simulink model "s12_euler_fvm_radiation_boundary_driver_ref"  (R2026a)
settings: Solver=FixedStepDiscrete  StartTime=0  StopTime=5.8309037900874641e-08  FixedStep=5.8309037900874641e-08
settings Model: Creator=Jovi  LastModifiedBy=Jovi

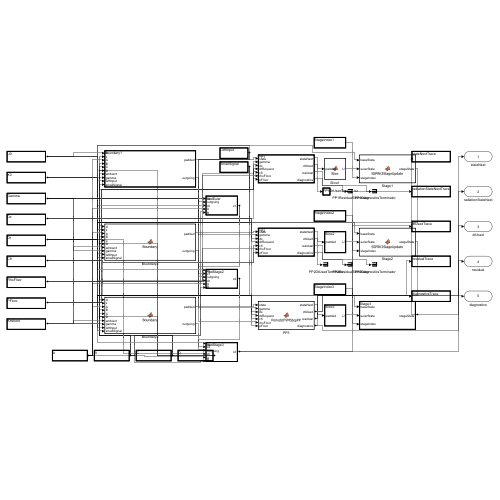
[thumbnail: Simulink's stored preview of the top-level diagram]
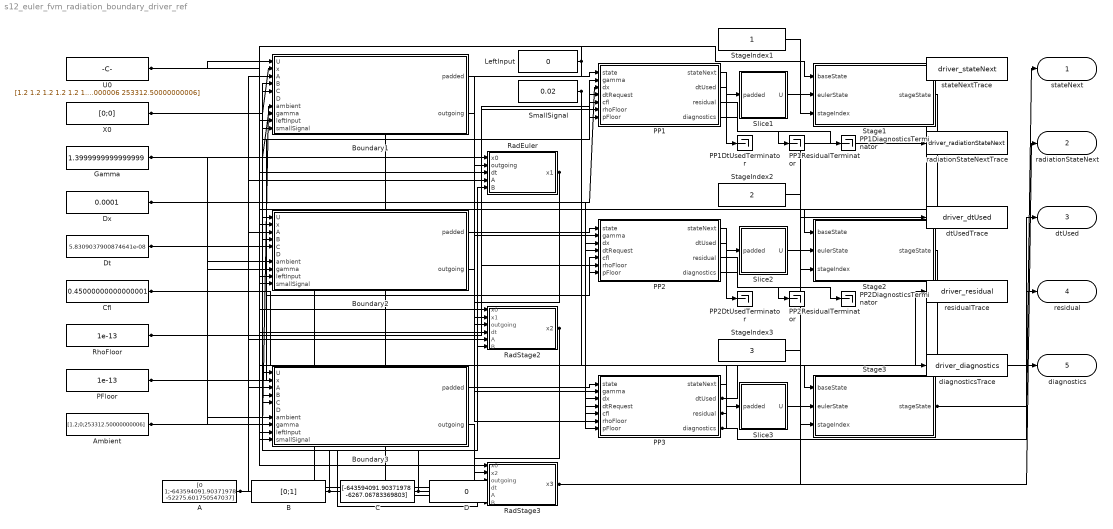
== system s12_euler_fvm_radiation_boundary_driver_ref ==
  A : Constant  Value=[0 1;-643594091.90371978 -52275.601750547037]  VectorParams1D=off  OutDataTypeStr=double
  Ambient : Constant  Value=[1.2;0;253312.50000000006]  VectorParams1D=off  OutDataTypeStr=double
  B : Constant  Value=[0;1]  VectorParams1D=off  OutDataTypeStr=double
  Boundary1 : MATLAB Function  TreatAsAtomicUnit=on
  Boundary2 : MATLAB Function  TreatAsAtomicUnit=on
  Boundary3 : MATLAB Function  TreatAsAtomicUnit=on
  C : Constant  Value=[-643594091.90371978 -6267.06783369803]  VectorParams1D=off  OutDataTypeStr=double
  Cfl : Constant  Value=0.45000000000000001  VectorParams1D=off  OutDataTypeStr=double
  D : Constant  Value=0  VectorParams1D=off  OutDataTypeStr=double
  Dt : Constant  Value=5.8309037900874641e-08  VectorParams1D=off  OutDataTypeStr=double
  Dx : Constant  Value=0.0001  VectorParams1D=off  OutDataTypeStr=double
  Gamma : Constant  Value=1.3999999999999999  VectorParams1D=off  OutDataTypeStr=double
  LeftInput : Constant  Value=0  VectorParams1D=off  OutDataTypeStr=double
  PFloor : Constant  Value=1e-13  VectorParams1D=off  OutDataTypeStr=double
  PP1 : MATLAB Function  TreatAsAtomicUnit=on
  PP1DiagnosticsTerminator : Terminator
  PP1DtUsedTerminator : Terminator
  PP1ResidualTerminator : Terminator
  PP2 : MATLAB Function  TreatAsAtomicUnit=on
  PP2DiagnosticsTerminator : Terminator
  PP2DtUsedTerminator : Terminator
  PP2ResidualTerminator : Terminator
  PP3 : MATLAB Function  TreatAsAtomicUnit=on
  RadEuler : MATLAB Function  TreatAsAtomicUnit=on
  RadStage2 : MATLAB Function  TreatAsAtomicUnit=on
  RadStage3 : MATLAB Function  TreatAsAtomicUnit=on
  RhoFloor : Constant  Value=1e-13  VectorParams1D=off  OutDataTypeStr=double
  Slice1 : MATLAB Function  TreatAsAtomicUnit=on
  Slice2 : MATLAB Function  TreatAsAtomicUnit=on
  Slice3 : MATLAB Function  TreatAsAtomicUnit=on
  SmallSignal : Constant  Value=0.02  VectorParams1D=off  OutDataTypeStr=double
  Stage1 : MATLAB Function  TreatAsAtomicUnit=on
  Stage2 : MATLAB Function  TreatAsAtomicUnit=on
  Stage3 : MATLAB Function  TreatAsAtomicUnit=on
  StageIndex1 : Constant  VectorParams1D=off  OutDataTypeStr=double
  StageIndex2 : Constant  Value=2  VectorParams1D=off  OutDataTypeStr=double
  StageIndex3 : Constant  Value=3  VectorParams1D=off  OutDataTypeStr=double
  U0 : Constant  Value=[1.2 1.2 1.2 1.2 1.2 1.2 1.2 1.2 1.2 1.2 1.2 1.2 1.2 1.2 1.2 1.2 1.2 1.2 1.2 1.2 1.2 1.2 1.2 1.2 1.2 1.2 1.2 1.2 1.2 1.2 1.2 1.2 1.2 1.2 1.2 1.2 1.2 1.2 1.2 1.2 1.2 1.2 1.2 1.2 1.2 1.2 1.2 1.2 1.2 1.2 1.2 1.2 1.2 1.2 1.2 1.2 1.2 1.2 1.2 1.2 1.2 1.2 1.2 1.2 1.2 1.2 1.2 1.2 1.2 1.2 1.2 1.2 1.2 1.2 1.2 1.2 1.2 1.2 1.2 1.2 1.2 1.2 1.2 1.2 1.2 1.2 1.2 1.2 1.2 1.2 1.2 1.2 1.2 1.2 1.2 1.2 1.2 1.2 1.2 1.2;0 0 0 0 0 0 0 0 0 0 0 0 0 0 0 0 0 0 0 0 0 0 0 0 0 0 0 0 0 0 0 0 0 0 0 0 0 0 0 0 0 0 0 0 0 0 0 0 0 0 0 0 0 0 0 0 0 0 0 0 0 0 0 0 0 0 0 0 0 0 0 0 0 0 0 0 0 0 0 0 0 0 0 0 0 0 0 0 0 0 0 0 0 0 0 0 0 0 0 0;253312.50000000006 253312.50000000006 253312.50000000006 253312.50000000006 253312.50000000006 253312.50000000006 253312.50000000006 253312.50000000006 253312.50000000006 253312.50000000006 253312.50000000006 253312.50000000006 253312.50000000006 253312.50000000006 253312.50000000006 253312.50000000006 253312.50000000006 253312.50000000006 253312.50000000006 253312.50000000006 253312.50000000006 253312.50000000006 253312.50000000006 253312.50000000006 253312.50000000006 253312.50000000006 253312.50000000006 253312.50000000006 253312.50000000006 253312.50000000006 253312.50000000006 253312.50000000006 253312.50000000006 253312.50000000006 253312.50000000006 253312.50000000006 253312.50000000006 253312.50000000006 253312.50000000006 253312.50000000006 253312.50000000006 253312.50000000006 253312.50000000006 253312.50000000006 253312.50000000006 253312.50000000006 253312.50000000006 253312.50000000006 253312.50000000006 253312.50000000006 253312.50000000006 253312.50000000006 253312.50000000006 253312.50000000006 253312.50000000006 253312.50000000006 253312.50000000006 253312.50000000006 253312.50000000006 253312.50000000006 253312.50000000006 253312.50000000006 253312.50000000006 253312.50000000006 253312.50000000006 253312.50000000006 253312.50000000006 253312.50000000006 253312.50000000006 253312.50000000006 253312.50000000006 253312.50000000006 253312.50000000006 253312.50000000006 253312.50000000006 253312.50000000006 253312.50000000006 253312.50000000006 253312.50000000006 253312.50000000006 253312.50000000006 253312.50000000006 253312.50000000006 253312.50000000006 253312.50000000006 253312.50000000006 253312.50000000006 253312.50000000006 253312.50000000006 253312.50000000006 253312.50000000006 253312.50000000006 253312.50000000006 253312.50000000006 253312.50000000006 253312.50000000006 253312.50000000006 253312.50000000006 253312.50000000006 253312.50000000006]  VectorParams1D=off  OutDataTypeStr=double
  X0 : Constant  Value=[0;0]  VectorParams1D=off  OutDataTypeStr=double
  diagnosticsTrace : ToWorkspace  VariableName=driver_diagnostics  SaveFormat=Structure With Time
      settings: MaxDataPoints=1
  dtUsedTrace : ToWorkspace  VariableName=driver_dtUsed  SaveFormat=Structure With Time
      settings: MaxDataPoints=1
  radiationStateNextTrace : ToWorkspace  VariableName=driver_radiationStateNext  SaveFormat=Structure With Time
      settings: MaxDataPoints=1
  residualTrace : ToWorkspace  VariableName=driver_residual  SaveFormat=Structure With Time
      settings: MaxDataPoints=1
  stateNextTrace : ToWorkspace  VariableName=driver_stateNext  SaveFormat=Structure With Time
      settings: MaxDataPoints=1
  stateNext : Outport
  radiationStateNext : Outport  Port=2
  dtUsed : Outport  Port=3
  residual : Outport  Port=4
  diagnostics : Outport  Port=5
  wires:
  U0/1 -> Boundary1/1(U), Stage1/1(baseState), Stage2/1(baseState), Stage3/1(baseState)
  X0/1 -> Boundary1/2(x), RadEuler/1(x0), RadStage2/1(x0), RadStage3/1(x0)
  A/1 -> Boundary1/3(A), RadEuler/4(A), Boundary2/3(A), RadStage2/5(A), Boundary3/3(A), RadStage3/5(A)
  B/1 -> Boundary1/4(B), RadEuler/5(B), Boundary2/4(B), RadStage2/6(B), Boundary3/4(B), RadStage3/6(B)
  C/1 -> Boundary1/5(C), Boundary2/5(C), Boundary3/5(C)
  D/1 -> Boundary1/6(D), Boundary2/6(D), Boundary3/6(D)
  Ambient/1 -> Boundary1/7(ambient), Boundary2/7(ambient), Boundary3/7(ambient)
  Gamma/1 -> Boundary1/8(gamma), PP1/2(gamma), Boundary2/8(gamma), PP2/2(gamma), Boundary3/8(gamma), PP3/2(gamma)
  LeftInput/1 -> Boundary1/9(leftInput), Boundary2/9(leftInput), Boundary3/9(leftInput)
  SmallSignal/1 -> Boundary1/10(smallSignal), Boundary2/10(smallSignal), Boundary3/10(smallSignal)
  Boundary1/1(padded) -> PP1/1(state)
  Dx/1 -> PP1/3(dx), PP2/3(dx), PP3/3(dx)
  Dt/1 -> PP1/4(dtRequest), RadEuler/3(dt), PP2/4(dtRequest), RadStage2/4(dt), PP3/4(dtRequest), RadStage3/4(dt)
  Cfl/1 -> PP1/5(cfl), PP2/5(cfl), PP3/5(cfl)
  RhoFloor/1 -> PP1/6(rhoFloor), PP2/6(rhoFloor), PP3/6(rhoFloor)
  PFloor/1 -> PP1/7(pFloor), PP2/7(pFloor), PP3/7(pFloor)
  PP1/1(stateNext) -> Slice1/1(padded)
  Slice1/1(U) -> Stage1/2(eulerState)
  StageIndex1/1 -> Stage1/3(stageIndex)
  Stage1/1(stageState) -> Boundary2/1(U)
  Boundary1/2(outgoing) -> RadEuler/2(outgoing)
  RadEuler/1(x1) -> Boundary2/2(x), RadStage2/2(x1)
  Boundary2/1(padded) -> PP2/1(state)
  PP2/1(stateNext) -> Slice2/1(padded)
  Slice2/1(U) -> Stage2/2(eulerState)
  StageIndex2/1 -> Stage2/3(stageIndex)
  Stage2/1(stageState) -> Boundary3/1(U)
  Boundary2/2(outgoing) -> RadStage2/3(outgoing)
  RadStage2/1(x2) -> Boundary3/2(x), RadStage3/2(x2)
  Boundary3/1(padded) -> PP3/1(state)
  PP3/1(stateNext) -> Slice3/1(padded)
  Slice3/1(U) -> Stage3/2(eulerState)
  StageIndex3/1 -> Stage3/3(stageIndex)
  Boundary3/2(outgoing) -> RadStage3/3(outgoing)
  Stage3/1(stageState) -> stateNext/1, stateNextTrace/1
  RadStage3/1(x3) -> radiationStateNext/1, radiationStateNextTrace/1
  PP3/2(dtUsed) -> dtUsed/1, dtUsedTrace/1
  PP3/3(residual) -> residual/1, residualTrace/1
  PP3/4(diagnostics) -> diagnostics/1, diagnosticsTrace/1
  PP1/2(dtUsed) -> PP1DtUsedTerminator/1
  PP1/3(residual) -> PP1ResidualTerminator/1
  PP1/4(diagnostics) -> PP1DiagnosticsTerminator/1
  PP2/2(dtUsed) -> PP2DtUsedTerminator/1
  PP2/3(residual) -> PP2ResidualTerminator/1
  PP2/4(diagnostics) -> PP2DiagnosticsTerminator/1

== matlab function s12_euler_fvm_radiation_boundary_driver_ref/Boundary2 ==
  data: U input; padded output; x input; A input; B input; C input; D input; ambient input; gamma input; leftInput input; smallSignal input; outgoing output
function [padded,outgoing] = Boundary(U,x,A,B,C,D,ambient,gamma,leftInput,smallSignal)
%#codegen
padded = zeros(3,size(U,2)+4); outgoing = 0;
[rho,u,p] = primitive(U(:,end),gamma); %#ok<ASGLU>
[rho0,u0,p0,c0] = primitive(ambient,gamma); %#ok<ASGLU>
outgoing = 0.5*((p-p0)+rho0*c0*u);
incoming = C*x + D*outgoing; perturbation = outgoing + incoming;
if max(abs([outgoing,incoming,perturbation])) > smallSignal*p0, error('S12:Driver:SmallSignal', 'Radiation boundary perturbation exceeds the configured small-signal limit.'); end
boundaryPressure = p0 + perturbation;
boundaryDensity = rho0 + perturbation/c0^2;
boundaryVelocity = (outgoing-incoming)/(rho0*c0);
right = conservative(boundaryDensity,boundaryVelocity,boundaryPressure,gamma);
left = leftBoundary(U(:,1),ambient,gamma,leftInput,smallSignal);
padded(:,1)=left; padded(:,2)=left; padded(:,3:end-2)=U; padded(:,end-1)=right; padded(:,end)=right;
end
function state = leftBoundary(interior,ambient,gamma,incomingPressure,smallSignal)
if all(interior == ambient), state=interior; return; end
[rho,u,p,c] = primitive(interior,gamma); [rho0,u0,p0,c0] = primitive(ambient,gamma);
if abs(incomingPressure) > smallSignal*p0, error('S12:Driver:SmallSignal', 'Radiation boundary perturbation exceeds the configured small-signal limit.'); end
if abs(incomingPressure) > 0
outgoing = 0.5*((p-p0)-rho0*c0*u); boundaryPressure=p0+incomingPressure+outgoing; boundaryVelocity=(incomingPressure-outgoing)/(rho0*c0); boundaryDensity=rho0*(boundaryPressure/p0)^(1/gamma);
else
incomingAmbient=u0+2*c0/(gamma-1); outgoing=u-2*c/(gamma-1); boundaryVelocity=0.5*(outgoing+incomingAmbient); boundarySoundSpeed=0.25*(gamma-1)*(incomingAmbient-outgoing); entropy=p/rho^gamma; boundaryDensity=(boundarySoundSpeed^2/(gamma*entropy))^(1/(gamma-1)); boundaryPressure=entropy*boundaryDensity^gamma;
end
state=conservative(boundaryDensity,boundaryVelocity,boundaryPressure,gamma);
end
function [rho,u,p,c] = primitive(state,gamma)
rho=state(1); u=state(2)/rho; p=(gamma-1)*(state(3)-0.5*rho*u^2); c=sqrt(gamma*p/rho);
end
function state=conservative(rho,u,p,gamma)
state=[rho;rho*u;p/(gamma-1)+0.5*rho*u^2];
end

== matlab function s12_euler_fvm_radiation_boundary_driver_ref/Boundary3 ==
  data: U input; padded output; x input; A input; B input; C input; D input; ambient input; gamma input; leftInput input; smallSignal input; outgoing output
function [padded,outgoing] = Boundary(U,x,A,B,C,D,ambient,gamma,leftInput,smallSignal)
%#codegen
padded = zeros(3,size(U,2)+4); outgoing = 0;
[rho,u,p] = primitive(U(:,end),gamma); %#ok<ASGLU>
[rho0,u0,p0,c0] = primitive(ambient,gamma); %#ok<ASGLU>
outgoing = 0.5*((p-p0)+rho0*c0*u);
incoming = C*x + D*outgoing; perturbation = outgoing + incoming;
if max(abs([outgoing,incoming,perturbation])) > smallSignal*p0, error('S12:Driver:SmallSignal', 'Radiation boundary perturbation exceeds the configured small-signal limit.'); end
boundaryPressure = p0 + perturbation;
boundaryDensity = rho0 + perturbation/c0^2;
boundaryVelocity = (outgoing-incoming)/(rho0*c0);
right = conservative(boundaryDensity,boundaryVelocity,boundaryPressure,gamma);
left = leftBoundary(U(:,1),ambient,gamma,leftInput,smallSignal);
padded(:,1)=left; padded(:,2)=left; padded(:,3:end-2)=U; padded(:,end-1)=right; padded(:,end)=right;
end
function state = leftBoundary(interior,ambient,gamma,incomingPressure,smallSignal)
if all(interior == ambient), state=interior; return; end
[rho,u,p,c] = primitive(interior,gamma); [rho0,u0,p0,c0] = primitive(ambient,gamma);
if abs(incomingPressure) > smallSignal*p0, error('S12:Driver:SmallSignal', 'Radiation boundary perturbation exceeds the configured small-signal limit.'); end
if abs(incomingPressure) > 0
outgoing = 0.5*((p-p0)-rho0*c0*u); boundaryPressure=p0+incomingPressure+outgoing; boundaryVelocity=(incomingPressure-outgoing)/(rho0*c0); boundaryDensity=rho0*(boundaryPressure/p0)^(1/gamma);
else
incomingAmbient=u0+2*c0/(gamma-1); outgoing=u-2*c/(gamma-1); boundaryVelocity=0.5*(outgoing+incomingAmbient); boundarySoundSpeed=0.25*(gamma-1)*(incomingAmbient-outgoing); entropy=p/rho^gamma; boundaryDensity=(boundarySoundSpeed^2/(gamma*entropy))^(1/(gamma-1)); boundaryPressure=entropy*boundaryDensity^gamma;
end
state=conservative(boundaryDensity,boundaryVelocity,boundaryPressure,gamma);
end
function [rho,u,p,c] = primitive(state,gamma)
rho=state(1); u=state(2)/rho; p=(gamma-1)*(state(3)-0.5*rho*u^2); c=sqrt(gamma*p/rho);
end
function state=conservative(rho,u,p,gamma)
state=[rho;rho*u;p/(gamma-1)+0.5*rho*u^2];
end

== matlab function s12_euler_fvm_radiation_boundary_driver_ref/Slice1 ==
  data: padded input; U output
function U = Slice(padded)
%#codegen
U=zeros(3,size(padded,2)-4); U(:,:)=padded(:,3:end-2);
end

== matlab function s12_euler_fvm_radiation_boundary_driver_ref/Slice2 ==
  data: padded input; U output
function U = Slice(padded)
%#codegen
U=zeros(3,size(padded,2)-4); U(:,:)=padded(:,3:end-2);
end

== matlab function s12_euler_fvm_radiation_boundary_driver_ref/Slice3 ==
  data: padded input; U output
function U = Slice(padded)
%#codegen
U=zeros(3,size(padded,2)-4); U(:,:)=padded(:,3:end-2);
end

== matlab function s12_euler_fvm_radiation_boundary_driver_ref/RadEuler ==
  data: x0 input; x1 output; outgoing input; dt input; A input; B input
function x1 = RadEuler(x0,outgoing,dt,A,B)
%#codegen
x1=zeros(2,1); x1=x0+dt*(A*x0+B*outgoing);
end

== matlab function s12_euler_fvm_radiation_boundary_driver_ref/PP2 ==
  data: state input; stateNext output; gamma input; dx input; dtRequest input; cfl input; dtUsed output; residual output; rhoFloor input; pFloor input; diagnostics output
function [stateNext,dtUsed,residual,diagnostics] = PeriodicFVMStepPP(state,gamma,dx,dtRequest,cfl,rhoFloor,pFloor)
%#codegen
validateState(state,gamma,rhoFloor,pFloor);
cellCount = size(state,2);
alphaStage = stageAlpha(state,gamma);
dtUsed = min(dtRequest,cfl*dx/alphaStage);
lambda = dtUsed/dx;
[rho,velocity,pressure] = recoverPrimitives(state,gamma);
slopeRho = minmodSlopes(rho);
slopeVelocity = minmodSlopes(velocity);
slopePressure = minmodSlopes(pressure);
leftPrimitive = zeros(3,cellCount);
rightPrimitive = zeros(3,cellCount);
minmodActivationCount = 0;
minmodLimitedCellCount = 0;
reconstructionPPActivationCount = 0;
reconstructionPPLimitedCellCount = 0;
reconstructionPPMinTheta = 1;
minimumReconstructedDensity = inf;
minimumReconstructedPressure = inf;
for cellIndex = 1:cellCount
    leftIndex = mod(cellIndex-2,cellCount)+1;
    rightIndex = mod(cellIndex,cellCount)+1;
    centered = 0.5*[rho(rightIndex)-rho(leftIndex);velocity(rightIndex)-velocity(leftIndex);pressure(rightIndex)-pressure(leftIndex)];
    slopes = [slopeRho(cellIndex);slopeVelocity(cellIndex);slopePressure(cellIndex)];
    limited = abs(slopes-centered) > 32*eps(max([1;abs(slopes);abs(centered)]));
    minmodActivationCount = minmodActivationCount + sum(limited);
    minmodLimitedCellCount = minmodLimitedCellCount + double(any(limited));
    primitive = [rho(cellIndex);velocity(cellIndex);pressure(cellIndex)];
    reconstruction = s12_pp_reconstruct_primitive(primitive,slopes,rhoFloor,pFloor);
    leftPrimitive(:,cellIndex) = reconstruction.left;
    rightPrimitive(:,cellIndex) = reconstruction.right;
    reconstructionPPMinTheta = min(reconstructionPPMinTheta,reconstruction.theta);
    active = reconstruction.theta < 1-32*eps;
    reconstructionPPActivationCount = reconstructionPPActivationCount + double(active);
    reconstructionPPLimitedCellCount = reconstructionPPLimitedCellCount + double(active);
    minimumReconstructedDensity = min(minimumReconstructedDensity,min(reconstruction.left(1),reconstruction.right(1)));
    minimumReconstructedPressure = min(minimumReconstructedPressure,min(reconstruction.left(3),reconstruction.right(3)));
end
interfaceFlux = zeros(3,cellCount);
fluxPPActivationCount = 0;
fluxPPLimitedInterfaceCount = 0;
fluxPPMinTheta = 1;
minimumAnchorDensity = inf;
minimumAnchorPressure = inf;
minimumFinalPartialDensity = inf;
minimumFinalPartialPressure = inf;
maximumFluxCorrectionNorm = 0;
for interfaceIndex = 1:cellCount
    rightIndex = mod(interfaceIndex,cellCount)+1;
    leftState = conservativeFromPrimitives(rightPrimitive(1,interfaceIndex),rightPrimitive(2,interfaceIndex),rightPrimitive(3,interfaceIndex),gamma);
    rightState = conservativeFromPrimitives(leftPrimitive(1,rightIndex),leftPrimitive(2,rightIndex),leftPrimitive(3,rightIndex),gamma);
    highFlux = hllcFlux(leftState,rightState,gamma);
    lowFlux = s12_pp_global_lf_flux(state(:,interfaceIndex),state(:,rightIndex),gamma,alphaStage);
    limitedFlux = s12_pp_limit_interface_flux(state(:,interfaceIndex),state(:,rightIndex),highFlux,lowFlux,lambda,gamma,rhoFloor,pFloor);
    interfaceFlux(:,interfaceIndex) = limitedFlux.flux;
    fluxPPMinTheta = min(fluxPPMinTheta,limitedFlux.theta);
    active = limitedFlux.theta < 1-32*eps;
    fluxPPActivationCount = fluxPPActivationCount + double(active);
    fluxPPLimitedInterfaceCount = fluxPPLimitedInterfaceCount + double(active);
    minimumAnchorDensity = min(minimumAnchorDensity,min(limitedFlux.low_left_partial(1),limitedFlux.low_right_partial(1)));
    minimumAnchorPressure = min(minimumAnchorPressure,min(pressureOf(limitedFlux.low_left_partial,gamma),pressureOf(limitedFlux.low_right_partial,gamma)));
    minimumFinalPartialDensity = min(minimumFinalPartialDensity,min(limitedFlux.left_partial(1),limitedFlux.right_partial(1)));
    minimumFinalPartialPressure = min(minimumFinalPartialPressure,min(pressureOf(limitedFlux.left_partial,gamma),pressureOf(limitedFlux.right_partial,gamma)));
    maximumFluxCorrectionNorm = max(maximumFluxCorrectionNorm,limitedFlux.correction_norm);
end
stateNext = zeros(size(state));
for cellIndex = 1:cellCount
    leftInterface = mod(cellIndex-2,cellCount)+1;
    stateNext(:,cellIndex) = state(:,cellIndex)-lambda*(interfaceFlux(:,cellIndex)-interfaceFlux(:,leftInterface));
end
validateState(stateNext,gamma,rhoFloor,pFloor);
residual = sum(stateNext-state,2).';
diagnostics = [minmodActivationCount,minmodLimitedCellCount,cellCount,reconstructionPPActivationCount,reconstructionPPLimitedCellCount,reconstructionPPMinTheta,minimumReconstructedDensity,minimumReconstructedPressure,0,fluxPPActivationCount,fluxPPLimitedInterfaceCount,cellCount,fluxPPMinTheta,minimumAnchorDensity,minimumAnchorPressure,minimumFinalPartialDensity,minimumFinalPartialPressure,alphaStage,maximumFluxCorrectionNorm,0];
end

function alpha = stageAlpha(state,gamma)
[rho,velocity,pressure] = recoverPrimitives(state,gamma);
alpha = max(abs(velocity)+sqrt(gamma*pressure./rho));
end

function validateState(state,gamma,rhoFloor,pFloor)
[rho,~,pressure] = recoverPrimitives(state,gamma);
if any(~isfinite(state(:))) || any(rho < rhoFloor) || any(pressure < pFloor)
    error('S12:Positivity:InvalidStage','A PP stage violated the configured floors.');
end
end

function [rho,velocity,pressure] = recoverPrimitives(state,gamma)
rho = state(1,:);
velocity = state(2,:)./rho;
pressure = (gamma-1)*(state(3,:)-0.5*rho.*velocity.^2);
end

function value = pressureOf(state,gamma)
rho = state(1);
velocity = state(2)/rho;
value = (gamma-1)*(state(3)-0.5*rho*velocity^2);
end

function state = conservativeFromPrimitives(rho,velocity,pressure,gamma)
state = [rho;rho*velocity;pressure/(gamma-1)+0.5*rho*velocity^2];
end

function slopes = minmodSlopes(values)
cellCount = numel(values);
slopes = zeros(size(values));
for cellIndex = 1:cellCount
    leftIndex = mod(cellIndex-2,cellCount)+1;
    rightIndex = mod(cellIndex,cellCount)+1;
    slopes(cellIndex) = minmod(values(cellIndex)-values(leftIndex),values(rightIndex)-values(cellIndex));
end
end

function value = minmod(leftDelta,rightDelta)
if leftDelta*rightDelta <= 0
    value = 0;
elseif abs(leftDelta) <= abs(rightDelta)
    value = leftDelta;
else
    value = rightDelta;
end
end

function flux = hllcFlux(stateL,stateR,gamma)
rhoL = stateL(1); rhoR = stateR(1);
uL = stateL(2)/rhoL; uR = stateR(2)/rhoR;
energyL = stateL(3); energyR = stateR(3);
pL = (gamma-1)*(energyL-0.5*rhoL*uL*uL);
pR = (gamma-1)*(energyR-0.5*rhoR*uR*uR);
soundL = sqrt(gamma*pL/rhoL); soundR = sqrt(gamma*pR/rhoR);
sL = min(uL-soundL,uR-soundR); sR = max(uL+soundL,uR+soundR);
sM = (pR-pL+rhoL*uL*(sL-uL)-rhoR*uR*(sR-uR))/(rhoL*(sL-uL)-rhoR*(sR-uR));
fluxL = [rhoL*uL;rhoL*uL*uL+pL;uL*(energyL+pL)];
fluxR = [rhoR*uR;rhoR*uR*uR+pR;uR*(energyR+pR)];
if sL >= 0
    flux = fluxL;
elseif sM >= 0
    rhoStarL = rhoL*(sL-uL)/(sL-sM);
    energyStarL = rhoStarL*(energyL/rhoL+(sM-uL)*(sM+pL/(rhoL*(sL-uL))));
    flux = fluxL+sL*([rhoStarL;rhoStarL*sM;energyStarL]-stateL);
elseif sR > 0
    rhoStarR = rhoR*(sR-uR)/(sR-sM);
    energyStarR = rhoStarR*(energyR/rhoR+(sM-uR)*(sM+pR/(rhoR*(sR-uR))));
    flux = fluxR+sR*([rhoStarR;rhoStarR*sM;energyStarR]-stateR);
else
    flux = fluxR;
end
end

== matlab function s12_euler_fvm_radiation_boundary_driver_ref/RadStage2 ==
  data: x0 input; x2 output; x1 input; outgoing input; dt input; A input; B input
function x2 = RadStage2(x0,x1,outgoing,dt,A,B)
%#codegen
x2=zeros(2,1); x2=0.75*x0+0.25*(x1+dt*(A*x1+B*outgoing));
end

== matlab function s12_euler_fvm_radiation_boundary_driver_ref/RadStage3 ==
  data: x0 input; x3 output; x2 input; outgoing input; dt input; A input; B input
function x3 = RadStage3(x0,x2,outgoing,dt,A,B)
%#codegen
x3=zeros(2,1); x3=(1/3)*x0+(2/3)*(x2+dt*(A*x2+B*outgoing));
end

== matlab function s12_euler_fvm_radiation_boundary_driver_ref/PP1 ==
  data: state input; stateNext output; gamma input; dx input; dtRequest input; cfl input; dtUsed output; residual output; rhoFloor input; pFloor input; diagnostics output
function [stateNext,dtUsed,residual,diagnostics] = PeriodicFVMStepPP(state,gamma,dx,dtRequest,cfl,rhoFloor,pFloor)
%#codegen
validateState(state,gamma,rhoFloor,pFloor);
cellCount = size(state,2);
alphaStage = stageAlpha(state,gamma);
dtUsed = min(dtRequest,cfl*dx/alphaStage);
lambda = dtUsed/dx;
[rho,velocity,pressure] = recoverPrimitives(state,gamma);
slopeRho = minmodSlopes(rho);
slopeVelocity = minmodSlopes(velocity);
slopePressure = minmodSlopes(pressure);
leftPrimitive = zeros(3,cellCount);
rightPrimitive = zeros(3,cellCount);
minmodActivationCount = 0;
minmodLimitedCellCount = 0;
reconstructionPPActivationCount = 0;
reconstructionPPLimitedCellCount = 0;
reconstructionPPMinTheta = 1;
minimumReconstructedDensity = inf;
minimumReconstructedPressure = inf;
for cellIndex = 1:cellCount
    leftIndex = mod(cellIndex-2,cellCount)+1;
    rightIndex = mod(cellIndex,cellCount)+1;
    centered = 0.5*[rho(rightIndex)-rho(leftIndex);velocity(rightIndex)-velocity(leftIndex);pressure(rightIndex)-pressure(leftIndex)];
    slopes = [slopeRho(cellIndex);slopeVelocity(cellIndex);slopePressure(cellIndex)];
    limited = abs(slopes-centered) > 32*eps(max([1;abs(slopes);abs(centered)]));
    minmodActivationCount = minmodActivationCount + sum(limited);
    minmodLimitedCellCount = minmodLimitedCellCount + double(any(limited));
    primitive = [rho(cellIndex);velocity(cellIndex);pressure(cellIndex)];
    reconstruction = s12_pp_reconstruct_primitive(primitive,slopes,rhoFloor,pFloor);
    leftPrimitive(:,cellIndex) = reconstruction.left;
    rightPrimitive(:,cellIndex) = reconstruction.right;
    reconstructionPPMinTheta = min(reconstructionPPMinTheta,reconstruction.theta);
    active = reconstruction.theta < 1-32*eps;
    reconstructionPPActivationCount = reconstructionPPActivationCount + double(active);
    reconstructionPPLimitedCellCount = reconstructionPPLimitedCellCount + double(active);
    minimumReconstructedDensity = min(minimumReconstructedDensity,min(reconstruction.left(1),reconstruction.right(1)));
    minimumReconstructedPressure = min(minimumReconstructedPressure,min(reconstruction.left(3),reconstruction.right(3)));
end
interfaceFlux = zeros(3,cellCount);
fluxPPActivationCount = 0;
fluxPPLimitedInterfaceCount = 0;
fluxPPMinTheta = 1;
minimumAnchorDensity = inf;
minimumAnchorPressure = inf;
minimumFinalPartialDensity = inf;
minimumFinalPartialPressure = inf;
maximumFluxCorrectionNorm = 0;
for interfaceIndex = 1:cellCount
    rightIndex = mod(interfaceIndex,cellCount)+1;
    leftState = conservativeFromPrimitives(rightPrimitive(1,interfaceIndex),rightPrimitive(2,interfaceIndex),rightPrimitive(3,interfaceIndex),gamma);
    rightState = conservativeFromPrimitives(leftPrimitive(1,rightIndex),leftPrimitive(2,rightIndex),leftPrimitive(3,rightIndex),gamma);
    highFlux = hllcFlux(leftState,rightState,gamma);
    lowFlux = s12_pp_global_lf_flux(state(:,interfaceIndex),state(:,rightIndex),gamma,alphaStage);
    limitedFlux = s12_pp_limit_interface_flux(state(:,interfaceIndex),state(:,rightIndex),highFlux,lowFlux,lambda,gamma,rhoFloor,pFloor);
    interfaceFlux(:,interfaceIndex) = limitedFlux.flux;
    fluxPPMinTheta = min(fluxPPMinTheta,limitedFlux.theta);
    active = limitedFlux.theta < 1-32*eps;
    fluxPPActivationCount = fluxPPActivationCount + double(active);
    fluxPPLimitedInterfaceCount = fluxPPLimitedInterfaceCount + double(active);
    minimumAnchorDensity = min(minimumAnchorDensity,min(limitedFlux.low_left_partial(1),limitedFlux.low_right_partial(1)));
    minimumAnchorPressure = min(minimumAnchorPressure,min(pressureOf(limitedFlux.low_left_partial,gamma),pressureOf(limitedFlux.low_right_partial,gamma)));
    minimumFinalPartialDensity = min(minimumFinalPartialDensity,min(limitedFlux.left_partial(1),limitedFlux.right_partial(1)));
    minimumFinalPartialPressure = min(minimumFinalPartialPressure,min(pressureOf(limitedFlux.left_partial,gamma),pressureOf(limitedFlux.right_partial,gamma)));
    maximumFluxCorrectionNorm = max(maximumFluxCorrectionNorm,limitedFlux.correction_norm);
end
stateNext = zeros(size(state));
for cellIndex = 1:cellCount
    leftInterface = mod(cellIndex-2,cellCount)+1;
    stateNext(:,cellIndex) = state(:,cellIndex)-lambda*(interfaceFlux(:,cellIndex)-interfaceFlux(:,leftInterface));
end
validateState(stateNext,gamma,rhoFloor,pFloor);
residual = sum(stateNext-state,2).';
diagnostics = [minmodActivationCount,minmodLimitedCellCount,cellCount,reconstructionPPActivationCount,reconstructionPPLimitedCellCount,reconstructionPPMinTheta,minimumReconstructedDensity,minimumReconstructedPressure,0,fluxPPActivationCount,fluxPPLimitedInterfaceCount,cellCount,fluxPPMinTheta,minimumAnchorDensity,minimumAnchorPressure,minimumFinalPartialDensity,minimumFinalPartialPressure,alphaStage,maximumFluxCorrectionNorm,0];
end

function alpha = stageAlpha(state,gamma)
[rho,velocity,pressure] = recoverPrimitives(state,gamma);
alpha = max(abs(velocity)+sqrt(gamma*pressure./rho));
end

function validateState(state,gamma,rhoFloor,pFloor)
[rho,~,pressure] = recoverPrimitives(state,gamma);
if any(~isfinite(state(:))) || any(rho < rhoFloor) || any(pressure < pFloor)
    error('S12:Positivity:InvalidStage','A PP stage violated the configured floors.');
end
end

function [rho,velocity,pressure] = recoverPrimitives(state,gamma)
rho = state(1,:);
velocity = state(2,:)./rho;
pressure = (gamma-1)*(state(3,:)-0.5*rho.*velocity.^2);
end

function value = pressureOf(state,gamma)
rho = state(1);
velocity = state(2)/rho;
value = (gamma-1)*(state(3)-0.5*rho*velocity^2);
end

function state = conservativeFromPrimitives(rho,velocity,pressure,gamma)
state = [rho;rho*velocity;pressure/(gamma-1)+0.5*rho*velocity^2];
end

function slopes = minmodSlopes(values)
cellCount = numel(values);
slopes = zeros(size(values));
for cellIndex = 1:cellCount
    leftIndex = mod(cellIndex-2,cellCount)+1;
    rightIndex = mod(cellIndex,cellCount)+1;
    slopes(cellIndex) = minmod(values(cellIndex)-values(leftIndex),values(rightIndex)-values(cellIndex));
end
end

function value = minmod(leftDelta,rightDelta)
if leftDelta*rightDelta <= 0
    value = 0;
elseif abs(leftDelta) <= abs(rightDelta)
    value = leftDelta;
else
    value = rightDelta;
end
end

function flux = hllcFlux(stateL,stateR,gamma)
rhoL = stateL(1); rhoR = stateR(1);
uL = stateL(2)/rhoL; uR = stateR(2)/rhoR;
energyL = stateL(3); energyR = stateR(3);
pL = (gamma-1)*(energyL-0.5*rhoL*uL*uL);
pR = (gamma-1)*(energyR-0.5*rhoR*uR*uR);
soundL = sqrt(gamma*pL/rhoL); soundR = sqrt(gamma*pR/rhoR);
sL = min(uL-soundL,uR-soundR); sR = max(uL+soundL,uR+soundR);
sM = (pR-pL+rhoL*uL*(sL-uL)-rhoR*uR*(sR-uR))/(rhoL*(sL-uL)-rhoR*(sR-uR));
fluxL = [rhoL*uL;rhoL*uL*uL+pL;uL*(energyL+pL)];
fluxR = [rhoR*uR;rhoR*uR*uR+pR;uR*(energyR+pR)];
if sL >= 0
    flux = fluxL;
elseif sM >= 0
    rhoStarL = rhoL*(sL-uL)/(sL-sM);
    energyStarL = rhoStarL*(energyL/rhoL+(sM-uL)*(sM+pL/(rhoL*(sL-uL))));
    flux = fluxL+sL*([rhoStarL;rhoStarL*sM;energyStarL]-stateL);
elseif sR > 0
    rhoStarR = rhoR*(sR-uR)/(sR-sM);
    energyStarR = rhoStarR*(energyR/rhoR+(sM-uR)*(sM+pR/(rhoR*(sR-uR))));
    flux = fluxR+sR*([rhoStarR;rhoStarR*sM;energyStarR]-stateR);
else
    flux = fluxR;
end
end

== matlab function s12_euler_fvm_radiation_boundary_driver_ref/PP3 ==
  data: state input; stateNext output; gamma input; dx input; dtRequest input; cfl input; dtUsed output; residual output; rhoFloor input; pFloor input; diagnostics output
function [stateNext,dtUsed,residual,diagnostics] = PeriodicFVMStepPP(state,gamma,dx,dtRequest,cfl,rhoFloor,pFloor)
%#codegen
validateState(state,gamma,rhoFloor,pFloor);
cellCount = size(state,2);
alphaStage = stageAlpha(state,gamma);
dtUsed = min(dtRequest,cfl*dx/alphaStage);
lambda = dtUsed/dx;
[rho,velocity,pressure] = recoverPrimitives(state,gamma);
slopeRho = minmodSlopes(rho);
slopeVelocity = minmodSlopes(velocity);
slopePressure = minmodSlopes(pressure);
leftPrimitive = zeros(3,cellCount);
rightPrimitive = zeros(3,cellCount);
minmodActivationCount = 0;
minmodLimitedCellCount = 0;
reconstructionPPActivationCount = 0;
reconstructionPPLimitedCellCount = 0;
reconstructionPPMinTheta = 1;
minimumReconstructedDensity = inf;
minimumReconstructedPressure = inf;
for cellIndex = 1:cellCount
    leftIndex = mod(cellIndex-2,cellCount)+1;
    rightIndex = mod(cellIndex,cellCount)+1;
    centered = 0.5*[rho(rightIndex)-rho(leftIndex);velocity(rightIndex)-velocity(leftIndex);pressure(rightIndex)-pressure(leftIndex)];
    slopes = [slopeRho(cellIndex);slopeVelocity(cellIndex);slopePressure(cellIndex)];
    limited = abs(slopes-centered) > 32*eps(max([1;abs(slopes);abs(centered)]));
    minmodActivationCount = minmodActivationCount + sum(limited);
    minmodLimitedCellCount = minmodLimitedCellCount + double(any(limited));
    primitive = [rho(cellIndex);velocity(cellIndex);pressure(cellIndex)];
    reconstruction = s12_pp_reconstruct_primitive(primitive,slopes,rhoFloor,pFloor);
    leftPrimitive(:,cellIndex) = reconstruction.left;
    rightPrimitive(:,cellIndex) = reconstruction.right;
    reconstructionPPMinTheta = min(reconstructionPPMinTheta,reconstruction.theta);
    active = reconstruction.theta < 1-32*eps;
    reconstructionPPActivationCount = reconstructionPPActivationCount + double(active);
    reconstructionPPLimitedCellCount = reconstructionPPLimitedCellCount + double(active);
    minimumReconstructedDensity = min(minimumReconstructedDensity,min(reconstruction.left(1),reconstruction.right(1)));
    minimumReconstructedPressure = min(minimumReconstructedPressure,min(reconstruction.left(3),reconstruction.right(3)));
end
interfaceFlux = zeros(3,cellCount);
fluxPPActivationCount = 0;
fluxPPLimitedInterfaceCount = 0;
fluxPPMinTheta = 1;
minimumAnchorDensity = inf;
minimumAnchorPressure = inf;
minimumFinalPartialDensity = inf;
minimumFinalPartialPressure = inf;
maximumFluxCorrectionNorm = 0;
for interfaceIndex = 1:cellCount
    rightIndex = mod(interfaceIndex,cellCount)+1;
    leftState = conservativeFromPrimitives(rightPrimitive(1,interfaceIndex),rightPrimitive(2,interfaceIndex),rightPrimitive(3,interfaceIndex),gamma);
    rightState = conservativeFromPrimitives(leftPrimitive(1,rightIndex),leftPrimitive(2,rightIndex),leftPrimitive(3,rightIndex),gamma);
    highFlux = hllcFlux(leftState,rightState,gamma);
    lowFlux = s12_pp_global_lf_flux(state(:,interfaceIndex),state(:,rightIndex),gamma,alphaStage);
    limitedFlux = s12_pp_limit_interface_flux(state(:,interfaceIndex),state(:,rightIndex),highFlux,lowFlux,lambda,gamma,rhoFloor,pFloor);
    interfaceFlux(:,interfaceIndex) = limitedFlux.flux;
    fluxPPMinTheta = min(fluxPPMinTheta,limitedFlux.theta);
    active = limitedFlux.theta < 1-32*eps;
    fluxPPActivationCount = fluxPPActivationCount + double(active);
    fluxPPLimitedInterfaceCount = fluxPPLimitedInterfaceCount + double(active);
    minimumAnchorDensity = min(minimumAnchorDensity,min(limitedFlux.low_left_partial(1),limitedFlux.low_right_partial(1)));
    minimumAnchorPressure = min(minimumAnchorPressure,min(pressureOf(limitedFlux.low_left_partial,gamma),pressureOf(limitedFlux.low_right_partial,gamma)));
    minimumFinalPartialDensity = min(minimumFinalPartialDensity,min(limitedFlux.left_partial(1),limitedFlux.right_partial(1)));
    minimumFinalPartialPressure = min(minimumFinalPartialPressure,min(pressureOf(limitedFlux.left_partial,gamma),pressureOf(limitedFlux.right_partial,gamma)));
    maximumFluxCorrectionNorm = max(maximumFluxCorrectionNorm,limitedFlux.correction_norm);
end
stateNext = zeros(size(state));
for cellIndex = 1:cellCount
    leftInterface = mod(cellIndex-2,cellCount)+1;
    stateNext(:,cellIndex) = state(:,cellIndex)-lambda*(interfaceFlux(:,cellIndex)-interfaceFlux(:,leftInterface));
end
validateState(stateNext,gamma,rhoFloor,pFloor);
residual = sum(stateNext-state,2).';
diagnostics = [minmodActivationCount,minmodLimitedCellCount,cellCount,reconstructionPPActivationCount,reconstructionPPLimitedCellCount,reconstructionPPMinTheta,minimumReconstructedDensity,minimumReconstructedPressure,0,fluxPPActivationCount,fluxPPLimitedInterfaceCount,cellCount,fluxPPMinTheta,minimumAnchorDensity,minimumAnchorPressure,minimumFinalPartialDensity,minimumFinalPartialPressure,alphaStage,maximumFluxCorrectionNorm,0];
end

function alpha = stageAlpha(state,gamma)
[rho,velocity,pressure] = recoverPrimitives(state,gamma);
alpha = max(abs(velocity)+sqrt(gamma*pressure./rho));
end

function validateState(state,gamma,rhoFloor,pFloor)
[rho,~,pressure] = recoverPrimitives(state,gamma);
if any(~isfinite(state(:))) || any(rho < rhoFloor) || any(pressure < pFloor)
    error('S12:Positivity:InvalidStage','A PP stage violated the configured floors.');
end
end

function [rho,velocity,pressure] = recoverPrimitives(state,gamma)
rho = state(1,:);
velocity = state(2,:)./rho;
pressure = (gamma-1)*(state(3,:)-0.5*rho.*velocity.^2);
end

function value = pressureOf(state,gamma)
rho = state(1);
velocity = state(2)/rho;
value = (gamma-1)*(state(3)-0.5*rho*velocity^2);
end

function state = conservativeFromPrimitives(rho,velocity,pressure,gamma)
state = [rho;rho*velocity;pressure/(gamma-1)+0.5*rho*velocity^2];
end

function slopes = minmodSlopes(values)
cellCount = numel(values);
slopes = zeros(size(values));
for cellIndex = 1:cellCount
    leftIndex = mod(cellIndex-2,cellCount)+1;
    rightIndex = mod(cellIndex,cellCount)+1;
    slopes(cellIndex) = minmod(values(cellIndex)-values(leftIndex),values(rightIndex)-values(cellIndex));
end
end

function value = minmod(leftDelta,rightDelta)
if leftDelta*rightDelta <= 0
    value = 0;
elseif abs(leftDelta) <= abs(rightDelta)
    value = leftDelta;
else
    value = rightDelta;
end
end

function flux = hllcFlux(stateL,stateR,gamma)
rhoL = stateL(1); rhoR = stateR(1);
uL = stateL(2)/rhoL; uR = stateR(2)/rhoR;
energyL = stateL(3); energyR = stateR(3);
pL = (gamma-1)*(energyL-0.5*rhoL*uL*uL);
pR = (gamma-1)*(energyR-0.5*rhoR*uR*uR);
soundL = sqrt(gamma*pL/rhoL); soundR = sqrt(gamma*pR/rhoR);
sL = min(uL-soundL,uR-soundR); sR = max(uL+soundL,uR+soundR);
sM = (pR-pL+rhoL*uL*(sL-uL)-rhoR*uR*(sR-uR))/(rhoL*(sL-uL)-rhoR*(sR-uR));
fluxL = [rhoL*uL;rhoL*uL*uL+pL;uL*(energyL+pL)];
fluxR = [rhoR*uR;rhoR*uR*uR+pR;uR*(energyR+pR)];
if sL >= 0
    flux = fluxL;
elseif sM >= 0
    rhoStarL = rhoL*(sL-uL)/(sL-sM);
    energyStarL = rhoStarL*(energyL/rhoL+(sM-uL)*(sM+pL/(rhoL*(sL-uL))));
    flux = fluxL+sL*([rhoStarL;rhoStarL*sM;energyStarL]-stateL);
elseif sR > 0
    rhoStarR = rhoR*(sR-uR)/(sR-sM);
    energyStarR = rhoStarR*(energyR/rhoR+(sM-uR)*(sM+pR/(rhoR*(sR-uR))));
    flux = fluxR+sR*([rhoStarR;rhoStarR*sM;energyStarR]-stateR);
else
    flux = fluxR;
end
end

== matlab function s12_euler_fvm_radiation_boundary_driver_ref/Stage1 ==
  data: baseState input; stageState output; eulerState input; stageIndex input
function stageState = SSPRK3StageUpdate(baseState,eulerState,stageIndex)
%#codegen
if stageIndex == 1
    stageState = eulerState;
elseif stageIndex == 2
    stageState = 0.75*baseState + 0.25*eulerState;
elseif stageIndex == 3
    stageState = (1.0/3.0)*baseState + (2.0/3.0)*eulerState;
else
    error('S12:SSPRK3:InvalidStage','stageIndex must be 1, 2, or 3.');
end
end

== matlab function s12_euler_fvm_radiation_boundary_driver_ref/Stage2 ==
  data: baseState input; stageState output; eulerState input; stageIndex input
function stageState = SSPRK3StageUpdate(baseState,eulerState,stageIndex)
%#codegen
if stageIndex == 1
    stageState = eulerState;
elseif stageIndex == 2
    stageState = 0.75*baseState + 0.25*eulerState;
elseif stageIndex == 3
    stageState = (1.0/3.0)*baseState + (2.0/3.0)*eulerState;
else
    error('S12:SSPRK3:InvalidStage','stageIndex must be 1, 2, or 3.');
end
end

== matlab function s12_euler_fvm_radiation_boundary_driver_ref/Stage3 ==
  data: baseState input; stageState output; eulerState input; stageIndex input
function stageState = SSPRK3StageUpdate(baseState,eulerState,stageIndex)
%#codegen
if stageIndex == 1
    stageState = eulerState;
elseif stageIndex == 2
    stageState = 0.75*baseState + 0.25*eulerState;
elseif stageIndex == 3
    stageState = (1.0/3.0)*baseState + (2.0/3.0)*eulerState;
else
    error('S12:SSPRK3:InvalidStage','stageIndex must be 1, 2, or 3.');
end
end

== matlab function s12_euler_fvm_radiation_boundary_driver_ref/Boundary1 ==
  data: U input; padded output; x input; A input; B input; C input; D input; ambient input; gamma input; leftInput input; smallSignal input; outgoing output
function [padded,outgoing] = Boundary(U,x,A,B,C,D,ambient,gamma,leftInput,smallSignal)
%#codegen
padded = zeros(3,size(U,2)+4); outgoing = 0;
[rho,u,p] = primitive(U(:,end),gamma); %#ok<ASGLU>
[rho0,u0,p0,c0] = primitive(ambient,gamma); %#ok<ASGLU>
outgoing = 0.5*((p-p0)+rho0*c0*u);
incoming = C*x + D*outgoing; perturbation = outgoing + incoming;
if max(abs([outgoing,incoming,perturbation])) > smallSignal*p0, error('S12:Driver:SmallSignal', 'Radiation boundary perturbation exceeds the configured small-signal limit.'); end
boundaryPressure = p0 + perturbation;
boundaryDensity = rho0 + perturbation/c0^2;
boundaryVelocity = (outgoing-incoming)/(rho0*c0);
right = conservative(boundaryDensity,boundaryVelocity,boundaryPressure,gamma);
left = leftBoundary(U(:,1),ambient,gamma,leftInput,smallSignal);
padded(:,1)=left; padded(:,2)=left; padded(:,3:end-2)=U; padded(:,end-1)=right; padded(:,end)=right;
end
function state = leftBoundary(interior,ambient,gamma,incomingPressure,smallSignal)
if all(interior == ambient), state=interior; return; end
[rho,u,p,c] = primitive(interior,gamma); [rho0,u0,p0,c0] = primitive(ambient,gamma);
if abs(incomingPressure) > smallSignal*p0, error('S12:Driver:SmallSignal', 'Radiation boundary perturbation exceeds the configured small-signal limit.'); end
if abs(incomingPressure) > 0
outgoing = 0.5*((p-p0)-rho0*c0*u); boundaryPressure=p0+incomingPressure+outgoing; boundaryVelocity=(incomingPressure-outgoing)/(rho0*c0); boundaryDensity=rho0*(boundaryPressure/p0)^(1/gamma);
else
incomingAmbient=u0+2*c0/(gamma-1); outgoing=u-2*c/(gamma-1); boundaryVelocity=0.5*(outgoing+incomingAmbient); boundarySoundSpeed=0.25*(gamma-1)*(incomingAmbient-outgoing); entropy=p/rho^gamma; boundaryDensity=(boundarySoundSpeed^2/(gamma*entropy))^(1/(gamma-1)); boundaryPressure=entropy*boundaryDensity^gamma;
end
state=conservative(boundaryDensity,boundaryVelocity,boundaryPressure,gamma);
end
function [rho,u,p,c] = primitive(state,gamma)
rho=state(1); u=state(2)/rho; p=(gamma-1)*(state(3)-0.5*rho*u^2); c=sqrt(gamma*p/rho);
end
function state=conservative(rho,u,p,gamma)
state=[rho;rho*u;p/(gamma-1)+0.5*rho*u^2];
end
